simulink model "bipedal_robot_CTRL2"  (R2020b)
settings: Solver=ode23  StartTime=0.0  StopTime=Tsim  MaxStep=0.01  RelTol=1e-3  AbsTol=1e-3  EnableMultiTasking=on
values from neighbouring files (symbols this model uses):
  g = 9.80665    [bipedal.m]
  Tfil = Ts*10    (= 0.01)    [bipedal.m]
  total_mass = mlist(1) + ll_mass + rl_mass    [bipedal.m]
  Ts = 1/fs    (= 0.001)    [bipedal.m]
undefined symbols (not defined in the file or in its folder): Base, ctrl_cfg_rem, Fdist, LefAnklePitch, LefAnkleRoll, LefHipPitch, LefHipRoll, LefHipYaw, LefKnee, pg_traj, RigAnklePitch, RigAnkleRoll, RigHipPitch, RigHipRoll, RigHipYaw, RigKnee, sim_floor, Tdist, VAR_DIST, X, Y, Z
libraries: sm_lib x56, biped_lib x39, nesl_utility x18, simulink x3, Contact_Forces_Lib x2, robotmaniplib x1
(part 1 of 4)
settings Model: Creator=Andraž  LastModifiedBy=Andraž
settings SolverCC: AutoScaleAbsTol=off  ZeroCrossAlgorithm=Adaptive
settings DataIOCC: LimitDataPoints=on  MaxDataPoints=10000
settings OptimizationCC: DefaultParameterBehavior=Inlined  EnhancedBackFolding=on  PassReuseOutputArgsThreshold=0  OptimizeBlockOrder=speed  DifferentSizesBufferReuse=on  OptimizationCustomize=off
settings DebuggingCC: IgnoredZcDiagnostic=none  ParameterTunabilityLossMsg=error  AllowSymbolicDim=off  SFUnexpectedBacktrackingDiag=warning  SFNoUnconditionalDefaultTransitionDiag=warning  SFExecutionAtInitializationDiag=none  ArithmeticOperatorsInVariantConditions=warning
settings SFSimCC: SimCustomHeaderCode="#include \"magdwick.h\""  SimUserSources=magdwick.c  SimUseLocalCustomCode=off  CustomCodeUndefinedFunction=UseInterfaceOnly
settings RTWCC: RTWUseLocalCustomCode=off
settings CodeAppCC: ForceParamTrailComments=on  OperatorAnnotations=on
settings GRTTargetCC: TargetLangStandard=C89/C90 (ANSI)
settings ConfigComp: CovMetricSettings=dw  CovSaveCumulativeToWorkspaceVar=on  CovSaveSingleToWorkspaceVar=on  CovExternalEMLEnable=off  CovSFcnEnable=off
settings SimscapeCC: SimscapeLogType=all  SimscapeLogSimulationStatistics=on  SimscapeLogDataHistory=10000
settings DiagnosticsConfigSet: SimMechanicsRigidlyBoundBlock=none  SimMechanicsJointTargetOverSpecification=none
settings ExplorerConfigSet: InternalSimMechanicsExplorerSettings="<ExplorerConfiguration><canonicalview>default</canonicalview><AnimationSetting><BasePlaybackSpeed>1.0</BasePlaybackSpeed><PlaybackSpeedFactor>1.0</PlaybackSpeedFactor></AnimationSetting><TilePanel><TileInfo><Tiles Columns=\"1\" Count=\"1\" Rows=\"1\"><Column Weight=\"1\"/><Row Weight=\"1\"/><Tile Height=\"1\" Width=\"1\" X=\"0\" Y=\"0\"/></Tiles></TileInfo><SceneInfo><SceneViewer><BGColor><R>0.921568632125854492</R><G>0.913725495338439941</G><B>0.929411768913269043</B></BGColor><Camera><DoPerspective>off</DoPerspective><Position><X>1.46613297561511291</X><Y>0.0453876523198907741</Y><Z>0.392041392879294182</Z></Position><Center><X>-5.43948861508880555e-08</X><Y>0.0453876523198907741</Y><Z>0.392041392879294182</Z></Center><Up><X>-0</X><Y>0</Y><Z>1</Z></Up><ViewLimDist>1</ViewLimDist><YLim>0.627694802072910396</YLim><XLim>0.478013733886293257</XLim></Camera></SceneViewer></SceneInfo></TilePanel><MechEditorPanel><Cameras/><GfxPanelCameraMap/><VideoCreator><PlaybackSpeedRatio>1.0</PlaybackSpeedRatio><FrameRate>30</FrameRate><VideoFormat>Motion JPEG AVI</VideoFormat><FrameSize>auto</FrameSize></VideoCreator></MechEditorPanel></ExplorerConfiguration>"

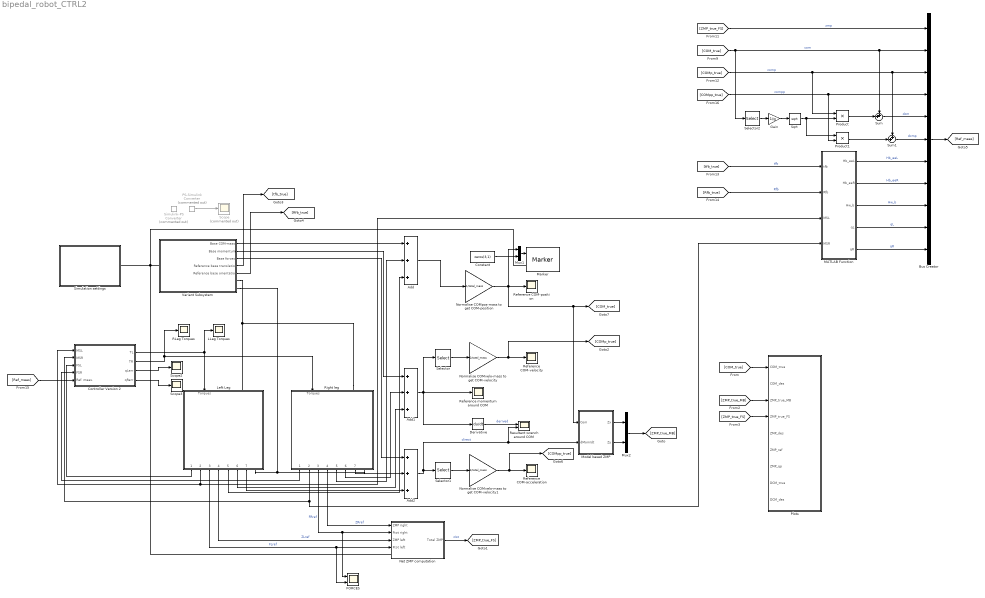
== system bipedal_robot_CTRL2 ==
  Add : Sum  Inputs=3
  Add1 : Sum  Inputs=3
  Add2 : Sum  Inputs=3
  Bus Creator : BusCreator  Inputs=11  OutDataTypeStr=Bus: meas_bus
  Constant : Constant  Value=zeros(3,1)
  Controller Version 2 : Subsystem  AncestorBlock=controller_lib/Controller Version 2  mask{ctrl_cfg_rem=ctrl_cfg_rem}
      mask prompts: ctrl_cfg_rem "Controller configuration structure"
  Derivative : Derivative  CoefficientInTFapproximation=400
  FORCES : Scope  NumInputPorts=2
  Gain : Gain  Gain=1/g
  LLeg Torques : Scope
  Left Leg : Subsystem
  MATLAB Function : MATLAB Function  TreatAsAtomicUnit=on  SystemSampleTime=Ts
  Marker : biped_lib/Marker  colour=[1.0 0.8 0.4]
  Model based ZMP : Subsystem  mask{M=total_mass, g=g, Tfil=Tfil*0.5}
      mask prompts: M "Mass"; g "Gravity"; Tfil "Filtering constant"
  Mux1 : Mux  Inputs=2
  Mux2 : Mux  Inputs=2
  Net ZMP computation : Subsystem
  Normalise COMpos-mass to get COM-position : Gain  Gain=1/total_mass
  Normalise COMvelo-mass to get COM-velocity : Gain  Gain=1/total_mass
  Normalise COMvelo-mass to get COM-velocity1 : Gain  Gain=1/total_mass
  PS-Simulink Converter : nesl_utility/PS-Simulink Converter  Commented=on  PhysicalDomain=network_engine_domain  SubClassName=ps_output  LeftPortType=input  RightPortType=output  PseudoPeriodic=off  Frequencies=[]  Unit=inherit  AffineConversion=off
      settings: SourceProductName=Utilities
  Plots : Subsystem
  Product : Product
  Product1 : Product
  RLeg Torques : Scope
  Reference COM-acceleration : Scope
  Reference COM-position : Scope
  Reference COM-velocity : Scope
  Reference momentum around COM : Scope
  Resultant wrench around COM : Scope  NumInputPorts=2
  Right leg : Subsystem
  Scope : Scope  Commented=on
  Scope2 : Scope
  Scope3 : Scope
  Selector : Selector  InputPortWidth=6  IndexOptions=Index vector (dialog)  Indices=[1 2 3]  OutputSizes=1
  Selector1 : Selector  InputPortWidth=6  IndexOptions=Index vector (dialog)  Indices=[1 2 3]  OutputSizes=1
  Selector2 : Selector  InputPortWidth=3  IndexOptions=Index vector (dialog)  Indices=[3]  OutputSizes=1
  Simulation settings : Subsystem
  Simulink-PS Converter : nesl_utility/Simulink-PS Converter  Commented=on  PhysicalDomain=network_engine_domain  SubClassName=ps_input  LeftPortType=input  RightPortType=output  PseudoPeriodic=off  Frequencies=[]  NoiseDistribution=none  NoiseParameters=[]  Unit=1  AffineConversion=off  FilteringAndDerivatives=provide  SimscapeFilterOrder=1  InputFilterTimeConstant=0.001  UdotUserProvided=0
      settings: SourceProductName=Utilities
  Sqrt : Sqrt  SaturateOnIntegerOverflow=on
  Sum : Sum  Inputs=++|
  Sum1 : Sum  Inputs=++|
  Variant Subsystem : Subsystem  Variant=on
  wires:
  PS-Simulink Converter/1 -> Scope/1
  Controller Version 2/1(TL) -> LLeg Torques/1, Left Leg/1(Torques)
  Controller Version 2/2(TR) -> Right leg/1(Torques), RLeg Torques/1
  Right leg/3(Total force) -> FORCES/1, Net ZMP computation/2(Ftot right)  "FRref"
  Left Leg/3(Total force) -> FORCES/2, Net ZMP computation/4(Ftot left)  "FLref"
  Right leg/4(Zero moment point) -> Net ZMP computation/1(ZMP right)  "ZRref"
  Left Leg/4(Zero moment point) -> Net ZMP computation/3(ZMP left)  "ZLref"
  Net ZMP computation/1(Total ZMP) -> [ZMP_true_FS]  "zIst"
  Left Leg/5(Leg COM-mass) -> Add/3
  Right leg/5(Leg COM-mass) -> Add/2
  Add/1 -> Normalise COMpos-mass to get COM-position/1
  Add1/1 -> Derivative/1, Reference momentum around COM/1, Selector/1
  Right leg/6(Leg momentum) -> Add1/2
  Left Leg/6(Leg momentum) -> Add1/3
  Derivative/1 -> Resultant wrench around COM/1  "derived"
  Selector/1 -> Normalise COMvelo-mass to get COM-velocity/1
  Normalise COMvelo-mass to get COM-velocity/1 -> [COMp_true], Reference COM-velocity/1
  Right leg/7(Leg momentum1) -> Add2/2
  Left Leg/7(Leg momentum1) -> Add2/3
  Add2/1 -> Selector1/1, Resultant wrench around COM/2, Model based ZMP/2(dMom/dt)  "direct"
  Normalise COMvelo-mass to get COM-velocity1/1 -> [COMpp_true], Reference COM-acceleration/1
  Selector1/1 -> Normalise COMvelo-mass to get COM-velocity1/1
  Normalise COMpos-mass to get COM-position/1 -> Mux1/1, Model based ZMP/1(Com), [COM_true], Reference COM-position/1
  Mux1/1 -> Marker/1
  Constant/1 -> Mux1/2
  Model based ZMP/1(Zx) -> Mux2/1
  Model based ZMP/2(Zy) -> Mux2/2
  Mux2/1 -> [ZMP_true_MB]
  [COM_true] -> Plots/1(COM_true)
  [ZMP_true_MB] -> Plots/3(ZMP_true_MB)
  [ZMP_true_FS] -> Plots/4(ZMP_true_FS)
  Left Leg/2(Motor sensory data) -> MATLAB Function/3(MSL), Controller Version 2/1(MSL)
  Right leg/2(Motor sensory data) -> MATLAB Function/4(MSR), Controller Version 2/2(MSR)
  Left Leg/1(Contact data) -> Controller Version 2/3(FSL)
  Right leg/1(Contact data) -> Controller Version 2/4(FSR)
  Controller Version 2/3(qLerr) -> Scope2/1
  Controller Version 2/4(qRerr) -> Scope3/1
  [COM_true] -> Selector2/1, Sum/1, Bus Creator/2  "com"
  Sum/1 -> Bus Creator/5  "dcm"
  [ZMP_true_FS] -> Bus Creator/1  "zmp"
  [COMp_true] -> Product/1, Bus Creator/3, Sum1/1  "comp"
  [tfb_true] -> MATLAB Function/1(tfb)  "tfb"
  [Rfb_true] -> MATLAB Function/2(Rfb)  "Rfb"
  Bus Creator/1 -> [Ref_meas]
  [Ref_meas] -> Controller Version 2/5(Ref. meas.)
  [COMpp_true] -> Product1/2, Bus Creator/4  "compp"
  Gain/1 -> Sqrt/1
  Selector2/1 -> Gain/1
  Sqrt/1 -> Product1/1, Product/2
  Product/1 -> Sum/2
  Product1/1 -> Sum1/2
  Sum1/1 -> Bus Creator/6  "dcmp"
  MATLAB Function/3(Hw_b) -> Bus Creator/9  "Hw_b"
  MATLAB Function/1(Hb_eeL) -> Bus Creator/7  "Hb_eeL"
  MATLAB Function/2(Hb_eeR) -> Bus Creator/8  "Hb_eeR"
  MATLAB Function/4(qL) -> Bus Creator/10  "qL"
  MATLAB Function/5(qR) -> Bus Creator/11  "qR"
  Variant Subsystem/1(Base COM-mass) -> Add/1
  Variant Subsystem/2(Base momentum) -> Add1/1
  Variant Subsystem/3(Base forces) -> Add2/1
  Variant Subsystem/4(Reference base translation) -> [tfb_true]
  Variant Subsystem/5(Reference base orientation) -> [Rfb_true]
  connections:
  Marker/LConn1 -- Simulation settings/RConn1 -- Variant Subsystem/LConn1 -- Net ZMP computation/LConn1
  Right leg/LConn1 -- Variant Subsystem/RConn1 -- Left Leg/LConn1
  Left Leg/RConn1 -- Right leg/RConn1 -- Variant Subsystem/RConn2

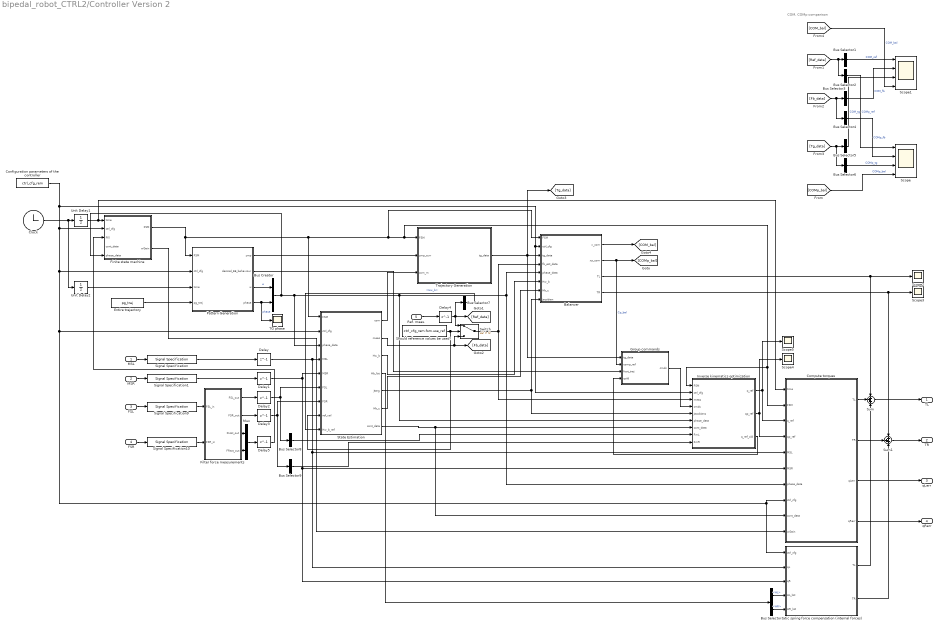
== system bipedal_robot_CTRL2/Controller Version 2 ==
  note: COM, COMp comparison
  MSL : Inport
  MSR : Inport  Port=2
  FSL : Inport  Port=3
  FSR : Inport  Port=4
  Ref. meas. : Inport  Port=5  OutDataTypeStr=Bus: meas_bus
  Balancer : MATLAB Function  TreatAsAtomicUnit=on
  Bus Creator : BusCreator  Inputs=2  OutDataTypeStr=Bus: ph_data_bus
  Bus Selector : BusSelector  OutputSignals=HL,HR
  Bus Selector1 : BusSelector  OutputSignals=com  OutputAsBus=on
  Bus Selector2 : BusSelector  OutputSignals=comp  OutputAsBus=on
  Bus Selector3 : BusSelector  OutputSignals=com  OutputAsBus=on
  Bus Selector4 : BusSelector  OutputSignals=comp  OutputAsBus=on
  Bus Selector5 : BusSelector  OutputSignals=com  OutputAsBus=on
  Bus Selector6 : BusSelector  OutputSignals=comp  OutputAsBus=on
  Bus Selector7 : BusSelector  OutputSignals=Hw_b
  Bus Selector8 : BusSelector  OutputSignals=Fm  OutputAsBus=on
  Bus Selector9 : BusSelector  OutputSignals=Fm  OutputAsBus=on
  Clock : Clock
  Compute torques : Subsystem
  Configuration parameters of the controller : Constant  Value=ctrl_cfg_rem  OutDataTypeStr=Bus: ctrl_cfg_rem_bus  SampleTime=ctrl_cfg_rem.par.Ts
  Delay : Delay  DelayLength=1  InitialCondition=ctrl_cfg_rem.fb_est.init.MSL  SampleTime=ctrl_cfg_rem.par.Ts
  Delay1 : Delay  DelayLength=1  InitialCondition=ctrl_cfg_rem.fb_est.init.MSR  SampleTime=ctrl_cfg_rem.par.Ts
  Delay2 : Delay  DelayLength=1  InitialCondition=ctrl_cfg_rem.fb_est.init.FSL  SampleTime=ctrl_cfg_rem.par.Ts
  Delay3 : Delay  DelayLength=1  InitialCondition=ctrl_cfg_rem.fb_est.init.FSR  SampleTime=ctrl_cfg_rem.par.Ts
  Delay4 : Delay  DelayLength=1  InitialCondition=0  SampleTime=ctrl_cfg_rem.par.Ts
  Delay5 : Delay  DelayLength=1  InitialCondition=[0;0]  SampleTime=ctrl_cfg_rem.par.Ts
  Entire trajectory : Constant  Value=pg_traj  VectorParams1D=off  OutDataTypeStr=Bus: pg_traj_bus  SampleTime=ctrl_cfg_rem.par.Ts
  Filter force measurements : Subsystem  mask{Tfil=ctrl_cfg_rem.fil.Tfil}
      mask prompts: Tfil "Filter T const"
  Finite state machine : MATLAB Function  TreatAsAtomicUnit=on
  Group commands : Subsystem
  Inverse kinematics optimization : Subsystem  Variant=on  mask{ik_opt=ctrl_cfg_rem.ik_opt, Ts=ctrl_cfg_rem.par.Ts}
      mask prompts: ik_opt "Ikine parameters"; Ts "Sampling time"
  Mux : Mux  Inputs=2
  Pattern Generation : Subsystem
  Scope : Scope  NumInputPorts=4
  Scope1 : Scope  NumInputPorts=4
  Scope{2..5} (4 alike) : Scope
  Should reference values be used? : Constant  Value=ctrl_cfg_rem.fsm.use_ref
  Signal Specification : SignalSpecification  OutDataTypeStr=Bus: leg_str_bus
  Signal Specification1 : SignalSpecification  OutDataTypeStr=Bus: leg_str_bus
  Signal Specification10 : SignalSpecification  OutDataTypeStr=Bus: fs_str_bus
  Signal Specification9 : SignalSpecification  OutDataTypeStr=Bus: fs_str_bus
  State Estimation : Subsystem  mask{fb_est=ctrl_cfg_rem.fb_est, Ts=ctrl_cfg_rem.par.Ts}
      mask prompts: fb_est "Floating base est. params"; Ts "Sampling time"
  Static spring force compensation (internal forces) : Subsystem
  Sum : Sum  Inputs=+++
  Sum1 : Sum  Inputs=+++
  Switch : Switch  Criteria=u2 > Threshold
  TG phase : Scope
  Trajectory Generation : Subsystem  Variant=on  mask{tg=ctrl_cfg_rem.tg}
      mask prompts: tg "Preview controller parameters"
  Unit Delay1 : UnitDelay  SampleTime=ctrl_cfg_rem.par.Ts  HasFrameUpgradeWarning=on
  Unit Delay2 : UnitDelay  SampleTime=ctrl_cfg_rem.par.Ts  HasFrameUpgradeWarning=on
  TL : Outport
  TR : Outport  Port=2
  qLerr : Outport  Port=3
  qRerr : Outport  Port=4
  wires:
  Compute torques/4(qRerr) -> qRerr/1
  Compute torques/3(qLerr) -> qLerr/1
  MSR/1 -> Signal Specification1/1
  FSL/1 -> Signal Specification9/1
  MSL/1 -> Signal Specification/1
  FSR/1 -> Signal Specification10/1
  Signal Specification1/1 -> Delay1/1
  Signal Specification/1 -> Delay/1
  Signal Specification9/1 -> Filter force measurements/1(FSL_in)
  Signal Specification10/1 -> Filter force measurements/2(FSR_in)
  Bus Selector/2 -> Static spring force compensation (internal forces)/5(HR_list)  "<HR>"
  Bus Selector/1 -> Static spring force compensation (internal forces)/4(HL_list)  "<HL>"
  Inverse kinematics optimization/3(q_ref_old) -> Group commands/4(qold)
  State Estimation/3(Hw_b) -> Balancer/6(Hw_b)
  Group commands/1(cmds) -> Inverse kinematics optimization/4(cmds)
  Pattern Generation/2(desired_EE_behaviour) -> Group commands/3(foot_traj)
  Trajectory Generation/1(tg_data) -> Group commands/1(tg_data), Balancer/3(tg_data), [Tg_data]
  Switch/1 -> Inverse kinematics optimization/3(meas), Balancer/4(fb_est_data)
  State Estimation/1(com) -> Trajectory Generation/3(com_m)
  Static spring force compensation (internal forces)/2(TR) -> Sum1/3
  Static spring force compensation (internal forces)/1(TL) -> Sum/3
  State Estimation/4(Hb_list) -> Bus Selector/1
  Compute torques/2(TR) -> Sum1/2
  Sum1/1 -> TR/1
  Sum/1 -> TL/1
  Compute torques/1(TL) -> Sum/2
  State Estimation/5(Jtarg) -> Balancer/8(jacobian), Inverse kinematics optimization/5(jacobians)
  Inverse kinematics optimization/2(qp_ref) -> Scope4/1, Compute torques/4(qp_ref)
  Inverse kinematics optimization/1(q_ref) -> Scope5/1, Compute torques/3(q_ref)
  Bus Creator/1 -> Finite state machine/5(phase_data), State Estimation/3(phase_data), Inverse kinematics optimization/6(phase_data), Balancer/5(phase_data), Compute torques/7(phase_data)
  Balancer/4(TR) -> Scope3/1, Sum1/1
  Balancer/3(TL) -> Scope2/1, Sum/1
  Pattern Generation/3(w) -> Bus Creator/1  "w"
  Delay2/1 -> State Estimation/6(FSL), Bus Selector8/1
  Unit Delay2/1 -> Pattern Generation/3(time)
  Finite state machine/1(FSM) -> Pattern Generation/1(FSM), Compute torques/2(FSM), Inverse kinematics optimization/1(FSM), Trajectory Generation/1(FSM), Balancer/1(FSM), State Estimation/1(FSM)
  Configuration parameters of the controller/1 -> Inverse kinematics optimization/2(ctrl_cfg), Balancer/2(ctrl_cfg), Pattern Generation/2(ctrl_cfg), State Estimation/2(ctrl_cfg), Static spring force compensation (internal forces)/1(ctrl_cfg), Compute torques/8(ctrl_cfg), Finite state machine/2(ctrl_cfg)
  Delay3/1 -> Bus Selector9/1, State Estimation/7(FSR)
  Delay1/1 -> State Estimation/5(MSR), Static spring force compensation (internal forces)/3(qR), Compute torques/6(MSR)
  Entire trajectory/1 -> Pattern Generation/4(pg_traj)
  Delay/1 -> Static spring force compensation (internal forces)/2(qL), Compute torques/5(MSL), State Estimation/4(MSL)
  Clock/1 -> Unit Delay2/1, Unit Delay1/1
  Unit Delay1/1 -> Compute torques/1(time), Finite state machine/1(time)
  Pattern Generation/4(phase) -> Bus Creator/2, TG phase/1  "phase"
  Pattern Generation/1(zmp) -> Trajectory Generation/2(zmp_curr)
  Balancer/2(xp_com) -> [COMp_bal], Group commands/2(comp_ref)  "Cp_bal"
  Ref. meas./1 -> Delay4/1
  Delay4/1 -> Bus Selector7/1, [Ref_data], Switch/1
  State Estimation/2(meas) -> [Fb_data], Switch/3
  Should reference values be used?/1 -> State Estimation/8(ref_val), Switch/2
  [Ref_data] -> Bus Selector2/1, Bus Selector1/1
  Bus Selector1/1 -> Scope1/1  "COM_ref"
  Bus Selector2/1 -> Scope/1  "COMp_ref"
  [Fb_data] -> Bus Selector4/1, Bus Selector3/1
  Bus Selector3/1 -> Scope1/2  "COM_fb"
  Bus Selector4/1 -> Scope/2  "COMp_fb"
  [COMp_bal] -> Scope/4  "COMp_bal"
  [Tg_data] -> Bus Selector6/1, Bus Selector5/1
  Bus Selector5/1 -> Scope1/3  "COM_tg"
  Bus Selector6/1 -> Scope/3  "COMp_tg"
  Balancer/1(x_com) -> [COM_bal]
  [COM_bal] -> Scope1/4  "COM_bal"
  Bus Selector7/1 -> State Estimation/9(Hw_b_ref)  "<Hw_b>"
  State Estimation/6(Hb_c) -> Balancer/7(Hb_c)
  Filter force measurements/1(FSL_out) -> Delay2/1
  Filter force measurements/2(FSR_out) -> Delay3/1
  Bus Selector8/1 -> Inverse kinematics optimization/8(FmL)
  Bus Selector9/1 -> Inverse kinematics optimization/9(FmR)
  Filter force measurements/4(FRtot_out) -> Mux/2
  Filter force measurements/3(FLtot_out) -> Mux/1
  Mux/1 -> Delay5/1
  State Estimation/7(cont_data) -> Compute torques/9(cont_data), Inverse kinematics optimization/7(cont_data)
  Delay5/1 -> Finite state machine/3(Ffil)
  Finite state machine/2(wGain) -> Compute torques/10(wGain)

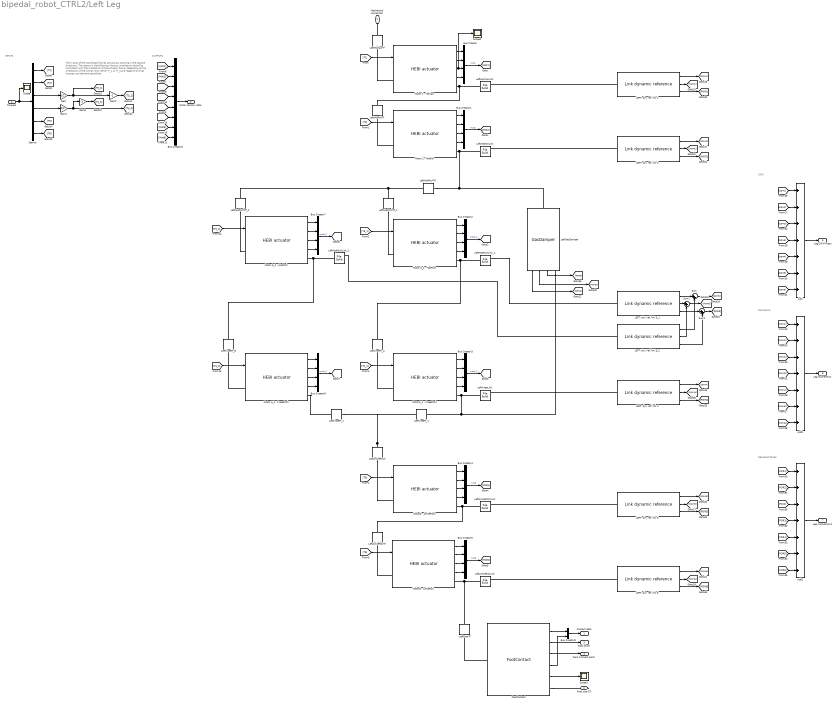
== system bipedal_robot_CTRL2/Left Leg ==
  note: Momentum
  note: COM
  note: OUTPUTS
  note: INPUTS
  note: The z-axes of the coordinate frames are always pointing in the
      | oposite directions. The reason is the following: the axis orientation
      | should be consistent with the orientation of the actuator frame. Depending on the orientation of the overall joint, either Ti_1 or Ti_2
      | are negative so that torques complement eachother
  note: Resultant forces
  Torques : Inport
  Add : Sum  Inputs=7
  Add1 : Sum  Inputs=7
  Add2 : Sum  Inputs=7
  Bus Creator{,1..5,7..8} (8 alike) : BusCreator  Inputs=4
  Bus Creator6 : BusCreator  Inputs=8  OutDataTypeStr=Bus: leg_str_bus
  Bus Creator9 : BusCreator  Inputs=2
  Demux : Demux  Outputs=6
  FootContact : biped_lib/FootContact  foot=foot  sim_floor=sim_floor  Ts=Ts
  Gain : Gain  Gain=1/2
  Gain1 : Gain  Gain=1/2
  Gain2 : Gain  Gain=-1
  Gain3 : Gain  Gain=-1
  LEFT: dyn. ref. link 1 : biped_lib/Link dynamic reference  M=LefHipYaw.body.com  I=LefHipYaw.body.inertia
  LEFT: dyn. ref. link 2 : biped_lib/Link dynamic reference  M=LefHipRoll.body.mass  I=LefHipRoll.body.inertia
  LEFT: dyn. ref. link 3_1 : biped_lib/Link dynamic reference  M=LefHipPitch.body.mass  I=LefHipPitch.body.inertia
  LEFT: dyn. ref. link 3_2 : biped_lib/Link dynamic reference  M=LefHipPitch.body.mass  I=LefHipPitch.body.inertia
  LEFT: dyn. ref. link 4 : biped_lib/Link dynamic reference  M=LefKnee.body.mass  I=LefKnee.body.inertia
  LEFT: dyn. ref. link 5 : biped_lib/Link dynamic reference  M=LefAnklePitch.body.mass  I=LefAnklePitch.body.inertia
  LEFT: dyn. ref. link 6 : biped_lib/Link dynamic reference  M=LefAnkleRoll.body.mass  I=LefAnkleRoll.body.inertia
  LeftAnklePitch : sm_lib/Frames and Transforms/Rigid Transform  TranslationMethod=Cartesian  TranslationStandardOffset=0  TranslationLengthUnit=m  TranslationStandardAxis=+Z  TranslationCartesianOffset=LefAnklePitch.pos  TranslationROffset=0  TranslationROffsetUnits=m  TranslationZOffset=0  TranslationZOffsetUnits=m  TranslationThetaOffset=0  TranslationThetaOffsetUnits=deg  RotationMethod=RotationSequence  RotationAngleUnits=deg  RotationStandardAxis=+Z  RotationAngle=0.0  RotationArbitraryAxis=[0 0 1]  FollAlignAxisA=+X  BaseAlignAxisA=+Y  FollAlignAxisB=+Y  BaseAlignAxisB=+Z  RotationSequenceAxes=FollowerAxes  RotationSequence=XYZ  RotationSequenceAngles=LefAnklePitch.rot  RotationSequenceAnglesUnits=rad  RotationMatrix=[1 0 0; 0 1 0; 0 0 1]
  LeftAnklePitchLink : sm_lib/Body Elements/File Solid  ExtGeomFileName=Link5L.stl  UnitType=Custom  ExtGeomFileUnits=mm  StepReaderType=HEX  ExportConvexHullGeometry=on  InertiaType=Custom  Mass=LefAnklePitch.body.mass  MassUnits=kg  CenterOfMass=LefAnklePitch.body.com  CenterOfMassUnits=m  MomentsOfInertia=LefAnklePitch.body.inertia(1:3)  MomentsOfInertiaUnits=kg*m^2  ProductsOfInertia=LefAnklePitch.body.inertia(4:6)  ProductsOfInertiaUnits=kg*m^2  BasedOnType=Mass  Density=1000  DensityUnits=kg/m^3  DoExposeReferenceFrame=on  SerializedFrames=<Frames><Frame><Id>Frame1</Id><Value><Name>COM</Name><Origin><Source>CenterOfMassFrame</Source><FeatureName></FeatureName></Origin><PrimaryAxis><DefinedDirection>+Z</DefinedDirection><Source>ReferenceFrame</Source><SourceDirection>+Z</SourceDirection><FeatureName></FeatureName></PrimaryAxis><SecondaryAxis><DefinedDirection>+X</DefinedDirection><Source>ReferenceFrame</Source><SourceDirection>+X</SourceDirection><FeatureName></FeatureName></SecondaryAxis></Value></Frame></Frames>  GraphicType=FromGeometry  MarkerShape=Sphere  MarkerSize=10  GraphicVisPropType=SimpleVisualProperties  GraphicDiffuseColor=[0.5 0.5 0.5]  GraphicSpecularColor=[0.5 0.5 0.5 1.0]  GraphicAmbientColor=[0.15 0.15 0.15 1.0]  GraphicEmissiveColor=[0.0 0.0 0.0 1.0]  GraphicShininess=75  GraphicOpacity=1.0
  LeftAnkleRollLink : sm_lib/Body Elements/File Solid  ExtGeomFileName=Link6.stl  UnitType=Custom  ExtGeomFileUnits=mm  StepReaderType=HEX  ExportConvexHullGeometry=on  InertiaType=Custom  Mass=LefAnkleRoll.body.mass  MassUnits=kg  CenterOfMass=LefAnkleRoll.body.com  CenterOfMassUnits=m  MomentsOfInertia=LefAnkleRoll.body.inertia(1:3)  MomentsOfInertiaUnits=kg*m^2  ProductsOfInertia=LefAnkleRoll.body.inertia(4:6)  ProductsOfInertiaUnits=kg*m^2  BasedOnType=Mass  Density=1000  DensityUnits=kg/m^3  DoExposeReferenceFrame=on  SerializedFrames=<Frames><Frame><Id>Frame1</Id><Value><Name>COM</Name><Origin><Source>CenterOfMassFrame</Source><FeatureName></FeatureName></Origin><PrimaryAxis><DefinedDirection>+Z</DefinedDirection><Source>ReferenceFrame</Source><SourceDirection>+Z</SourceDirection><FeatureName></FeatureName></PrimaryAxis><SecondaryAxis><DefinedDirection>+X</DefinedDirection><Source>ReferenceFrame</Source><SourceDirection>+X</SourceDirection><FeatureName></FeatureName></SecondaryAxis></Value></Frame></Frames>  GraphicType=FromGeometry  MarkerShape=Sphere  MarkerSize=10  GraphicVisPropType=SimpleVisualProperties  GraphicDiffuseColor=[0.5 0.5 0.5]  GraphicSpecularColor=[0.5 0.5 0.5 1.0]  GraphicAmbientColor=[0.15 0.15 0.15 1.0]  GraphicEmissiveColor=[0.0 0.0 0.0 1.0]  GraphicShininess=75  GraphicOpacity=1.0
  LeftAnkleRollTf : sm_lib/Frames and Transforms/Rigid Transform  TranslationMethod=Cartesian  TranslationStandardOffset=0  TranslationLengthUnit=m  TranslationStandardAxis=+Z  TranslationCartesianOffset=LefAnkleRoll.pos  TranslationROffset=0  TranslationROffsetUnits=m  TranslationZOffset=0  TranslationZOffsetUnits=m  TranslationThetaOffset=0  TranslationThetaOffsetUnits=deg  RotationMethod=RotationSequence  RotationAngleUnits=deg  RotationStandardAxis=+Z  RotationAngle=0.0  RotationArbitraryAxis=[0 0 1]  FollAlignAxisA=+Z  BaseAlignAxisA=+X  FollAlignAxisB=+Y  BaseAlignAxisB=+Y  RotationSequenceAxes=FollowerAxes  RotationSequence=XYZ  RotationSequenceAngles=LefAnkleRoll.rot  RotationSequenceAnglesUnits=rad  RotationMatrix=[1 0 0; 0 1 0; 0 0 1]
  LeftFootTf : sm_lib/Frames and Transforms/Rigid Transform  TranslationMethod=Cartesian  TranslationStandardOffset=0  TranslationLengthUnit=m  TranslationStandardAxis=+Z  TranslationCartesianOffset=LefFoot.pos  TranslationROffset=0  TranslationROffsetUnits=m  TranslationZOffset=0  TranslationZOffsetUnits=m  TranslationThetaOffset=0  TranslationThetaOffsetUnits=deg  RotationMethod=RotationSequence  RotationAngleUnits=deg  RotationStandardAxis=+Z  RotationAngle=0.0  RotationArbitraryAxis=[0 0 1]  FollAlignAxisA=+Z  BaseAlignAxisA=+Y  FollAlignAxisB=+X  BaseAlignAxisB=+X  RotationSequenceAxes=FollowerAxes  RotationSequence=XYZ  RotationSequenceAngles=LefFoot.rot  RotationSequenceAnglesUnits=rad  RotationMatrix=[1 0 0; 0 1 0; 0 0 1]
  LeftGasDamper : biped_lib/GasDamper  mech=LefDamper
  LeftHipPitchLink_1 : sm_lib/Body Elements/File Solid  ExtGeomFileName=Link3.stl  UnitType=Custom  ExtGeomFileUnits=mm  StepReaderType=HEX  ExportConvexHullGeometry=on  InertiaType=Custom  Mass=LefHipPitch.body.mass  MassUnits=kg  CenterOfMass=LefHipPitch.body.com  CenterOfMassUnits=m  MomentsOfInertia=LefHipPitch.body.inertia(1:3)  MomentsOfInertiaUnits=kg*m^2  ProductsOfInertia=LefHipPitch.body.inertia(4:6)  ProductsOfInertiaUnits=kg*m^2  BasedOnType=Mass  Density=1000  DensityUnits=kg/m^3  DoExposeReferenceFrame=on  SerializedFrames=<Frames><Frame><Id>Frame1</Id><Value><Name>COM</Name><Origin><Source>CenterOfMassFrame</Source><FeatureName></FeatureName></Origin><PrimaryAxis><DefinedDirection>+Z</DefinedDirection><Source>ReferenceFrame</Source><SourceDirection>+Z</SourceDirection><FeatureName></FeatureName></PrimaryAxis><SecondaryAxis><DefinedDirection>+X</DefinedDirection><Source>ReferenceFrame</Source><SourceDirection>+X</SourceDirection><FeatureName></FeatureName></SecondaryAxis></Value></Frame></Frames>  GraphicType=FromGeometry  MarkerShape=Sphere  MarkerSize=10  GraphicVisPropType=SimpleVisualProperties  GraphicDiffuseColor=[0.5 0.5 0.5]  GraphicSpecularColor=[0.5 0.5 0.5 1.0]  GraphicAmbientColor=[0.15 0.15 0.15 1.0]  GraphicEmissiveColor=[0.0 0.0 0.0 1.0]  GraphicShininess=75  GraphicOpacity=1.0
  LeftHipPitchLink_2 : sm_lib/Body Elements/File Solid  ExtGeomFileName=Link3.stl  UnitType=Custom  ExtGeomFileUnits=mm  StepReaderType=HEX  ExportConvexHullGeometry=on  InertiaType=Custom  Mass=LefHipPitch.body.mass  MassUnits=kg  CenterOfMass=LefHipPitch.body.com  CenterOfMassUnits=m  MomentsOfInertia=LefHipPitch.body.inertia(1:3)  MomentsOfInertiaUnits=kg*m^2  ProductsOfInertia=LefHipPitch.body.inertia(4:6)  ProductsOfInertiaUnits=kg*m^2  BasedOnType=Mass  Density=1000  DensityUnits=kg/m^3  DoExposeReferenceFrame=on  SerializedFrames=<Frames><Frame><Id>Frame1</Id><Value><Name>COM</Name><Origin><Source>CenterOfMassFrame</Source><FeatureName></FeatureName></Origin><PrimaryAxis><DefinedDirection>+Z</DefinedDirection><Source>ReferenceFrame</Source><SourceDirection>+Z</SourceDirection><FeatureName></FeatureName></PrimaryAxis><SecondaryAxis><DefinedDirection>+X</DefinedDirection><Source>ReferenceFrame</Source><SourceDirection>+X</SourceDirection><FeatureName></FeatureName></SecondaryAxis></Value></Frame></Frames>  GraphicType=FromGeometry  MarkerShape=Sphere  MarkerSize=10  GraphicVisPropType=SimpleVisualProperties  GraphicDiffuseColor=[0.5 0.5 0.5]  GraphicSpecularColor=[0.5 0.5 0.5 1.0]  GraphicAmbientColor=[0.15 0.15 0.15 1.0]  GraphicEmissiveColor=[0.0 0.0 0.0 1.0]  GraphicShininess=75  GraphicOpacity=1.0
  LeftHipPitchTf : sm_lib/Frames and Transforms/Rigid Transform  TranslationMethod=Cartesian  TranslationStandardOffset=0  TranslationLengthUnit=m  TranslationStandardAxis=+Z  TranslationCartesianOffset=LefHipPitch.pos  TranslationROffset=0  TranslationROffsetUnits=m  TranslationZOffset=0  TranslationZOffsetUnits=m  TranslationThetaOffset=0  TranslationThetaOffsetUnits=deg  RotationMethod=RotationSequence  RotationAngleUnits=deg  RotationStandardAxis=+Z  RotationAngle=0.0  RotationArbitraryAxis=[0 0 1]  FollAlignAxisA=+Z  BaseAlignAxisA=-X  FollAlignAxisB=+Y  BaseAlignAxisB=+Y  RotationSequenceAxes=FollowerAxes  RotationSequence=XYZ  RotationSequenceAngles=LefHipPitch.rot  RotationSequenceAnglesUnits=rad  RotationMatrix=[1 0 0; 0 1 0; 0 0 1]
  LeftHipPitchTf_1 : sm_lib/Frames and Transforms/Rigid Transform  TranslationMethod=Cartesian  TranslationStandardOffset=0  TranslationLengthUnit=m  TranslationStandardAxis=+Z  TranslationCartesianOffset=LefHipPitch.pos_1  TranslationROffset=0  TranslationROffsetUnits=m  TranslationZOffset=0  TranslationZOffsetUnits=m  TranslationThetaOffset=0  TranslationThetaOffsetUnits=deg  RotationMethod=RotationSequence  RotationAngleUnits=deg  RotationStandardAxis=+Z  RotationAngle=0.0  RotationArbitraryAxis=[0 0 1]  FollAlignAxisA=+X  BaseAlignAxisA=+Y  FollAlignAxisB=+Y  BaseAlignAxisB=+Z  RotationSequenceAxes=FollowerAxes  RotationSequence=XYZ  RotationSequenceAngles=LefHipPitch.rot_1  RotationSequenceAnglesUnits=rad  RotationMatrix=[1 0 0; 0 1 0; 0 0 1]
  LeftHipPitchTf_2 : sm_lib/Frames and Transforms/Rigid Transform  TranslationMethod=Cartesian  TranslationStandardOffset=0  TranslationLengthUnit=m  TranslationStandardAxis=+Z  TranslationCartesianOffset=LefHipPitch.pos_2  TranslationROffset=0  TranslationROffsetUnits=m  TranslationZOffset=0  TranslationZOffsetUnits=m  TranslationThetaOffset=0  TranslationThetaOffsetUnits=deg  RotationMethod=RotationSequence  RotationAngleUnits=deg  RotationStandardAxis=+Z  RotationAngle=0.0  RotationArbitraryAxis=[0 0 1]  FollAlignAxisA=+X  BaseAlignAxisA=+Y  FollAlignAxisB=+Y  BaseAlignAxisB=+Z  RotationSequenceAxes=FollowerAxes  RotationSequence=XYZ  RotationSequenceAngles=LefHipPitch.rot_2  RotationSequenceAnglesUnits=rad  RotationMatrix=[1 0 0; 0 1 0; 0 0 1]
  LeftHipRollLink : sm_lib/Body Elements/File Solid  ExtGeomFileName=Link2.stl  UnitType=Custom  ExtGeomFileUnits=mm  StepReaderType=HEX  ExportConvexHullGeometry=on  InertiaType=Custom  Mass=LefHipRoll.body.mass  MassUnits=kg  CenterOfMass=LefHipRoll.body.com  CenterOfMassUnits=m  MomentsOfInertia=LefHipRoll.body.inertia(1:3)  MomentsOfInertiaUnits=kg*m^2  ProductsOfInertia=LefHipRoll.body.inertia(4:6)  ProductsOfInertiaUnits=kg*m^2  BasedOnType=Mass  Density=1000  DensityUnits=kg/m^3  DoExposeReferenceFrame=on  SerializedFrames=<Frames><Frame><Id>Frame1</Id><Value><Name>COM</Name><Origin><Source>CenterOfMassFrame</Source><FeatureName></FeatureName></Origin><PrimaryAxis><DefinedDirection>+Z</DefinedDirection><Source>ReferenceFrame</Source><SourceDirection>+Z</SourceDirection><FeatureName></FeatureName></PrimaryAxis><SecondaryAxis><DefinedDirection>+X</DefinedDirection><Source>ReferenceFrame</Source><SourceDirection>+X</SourceDirection><FeatureName></FeatureName></SecondaryAxis></Value></Frame></Frames>  GraphicType=FromGeometry  MarkerShape=Sphere  MarkerSize=10  GraphicVisPropType=SimpleVisualProperties  GraphicDiffuseColor=[0.5 0.5 0.5]  GraphicSpecularColor=[0.5 0.5 0.5 1.0]  GraphicAmbientColor=[0.15 0.15 0.15 1.0]  GraphicEmissiveColor=[0.0 0.0 0.0 1.0]  GraphicShininess=75  GraphicOpacity=1.0
  LeftHipRollTf : sm_lib/Frames and Transforms/Rigid Transform  TranslationMethod=Cartesian  TranslationStandardOffset=0  TranslationLengthUnit=m  TranslationStandardAxis=+Z  TranslationCartesianOffset=LefHipRoll.pos  TranslationROffset=0  TranslationROffsetUnits=m  TranslationZOffset=0  TranslationZOffsetUnits=m  TranslationThetaOffset=0  TranslationThetaOffsetUnits=deg  RotationMethod=RotationSequence  RotationAngleUnits=deg  RotationStandardAxis=+Z  RotationAngle=0.0  RotationArbitraryAxis=[0 0 1]  FollAlignAxisA=+Z  BaseAlignAxisA=+Y  FollAlignAxisB=+X  BaseAlignAxisB=+X  RotationSequenceAxes=FollowerAxes  RotationSequence=XYZ  RotationSequenceAngles=LefHipRoll.rot  RotationSequenceAnglesUnits=rad  RotationMatrix=[1 0 0; 0 1 0; 0 0 1]
  LeftHipYawLink : sm_lib/Body Elements/File Solid  ExtGeomFileName=Link1L.stl  UnitType=Custom  ExtGeomFileUnits=mm  StepReaderType=HEX  ExportConvexHullGeometry=on  InertiaType=Custom  Mass=LefHipYaw.body.mass  MassUnits=kg  CenterOfMass=LefHipYaw.body.com  CenterOfMassUnits=m  MomentsOfInertia=LefHipYaw.body.inertia(1:3)  MomentsOfInertiaUnits=kg*m^2  ProductsOfInertia=LefHipYaw.body.inertia(4:6)  ProductsOfInertiaUnits=kg*m^2  BasedOnType=Mass  Density=1000  DensityUnits=kg/m^3  DoExposeReferenceFrame=on  SerializedFrames=<Frames><Frame><Id>Frame1</Id><Value><Name>COM</Name><Origin><Source>CenterOfMassFrame</Source><FeatureName></FeatureName></Origin><PrimaryAxis><DefinedDirection>+Z</DefinedDirection><Source>ReferenceFrame</Source><SourceDirection>+Z</SourceDirection><FeatureName></FeatureName></PrimaryAxis><SecondaryAxis><DefinedDirection>+X</DefinedDirection><Source>ReferenceFrame</Source><SourceDirection>+X</SourceDirection><FeatureName></FeatureName></SecondaryAxis></Value></Frame></Frames>  GraphicType=FromGeometry  MarkerShape=Sphere  MarkerSize=10  GraphicVisPropType=SimpleVisualProperties  GraphicDiffuseColor=[0.5 0.5 0.5]  GraphicSpecularColor=[0.5 0.5 0.5 1.0]  GraphicAmbientColor=[0.15 0.15 0.15 1.0]  GraphicEmissiveColor=[0.0 0.0 0.0 1.0]  GraphicShininess=75  GraphicOpacity=1.0
  LeftHipYawTf : sm_lib/Frames and Transforms/Rigid Transform  TranslationMethod=Cartesian  TranslationStandardOffset=0  TranslationLengthUnit=m  TranslationStandardAxis=+Z  TranslationCartesianOffset=LefHipYaw.pos  TranslationROffset=0  TranslationROffsetUnits=m  TranslationZOffset=0  TranslationZOffsetUnits=m  TranslationThetaOffset=0  TranslationThetaOffsetUnits=deg  RotationMethod=RotationSequence  RotationAngleUnits=deg  RotationStandardAxis=+Z  RotationAngle=0.0  RotationArbitraryAxis=[0 0 1]  FollAlignAxisA=+X  BaseAlignAxisA=+Y  FollAlignAxisB=+Y  BaseAlignAxisB=+Z  RotationSequenceAxes=FollowerAxes  RotationSequence=XYZ  RotationSequenceAngles=LefHipYaw.rot  RotationSequenceAnglesUnits=rad  RotationMatrix=[1 0 0; 0 1 0; 0 0 1]
  LeftKneeLink : sm_lib/Body Elements/File Solid  ExtGeomFileName=Link4.stl  UnitType=Custom  ExtGeomFileUnits=mm  StepReaderType=HEX  ExportConvexHullGeometry=on  InertiaType=Custom  Mass=LefKnee.body.mass  MassUnits=kg  CenterOfMass=LefKnee.body.com  CenterOfMassUnits=m  MomentsOfInertia=LefKnee.body.inertia(1:3)  MomentsOfInertiaUnits=kg*m^2  ProductsOfInertia=LefKnee.body.inertia(4:6)  ProductsOfInertiaUnits=kg*m^2  BasedOnType=Mass  Density=1000  DensityUnits=kg/m^3  DoExposeReferenceFrame=on  SerializedFrames=<Frames><Frame><Id>Frame1</Id><Value><Name>COM</Name><Origin><Source>CenterOfMassFrame</Source><FeatureName></FeatureName></Origin><PrimaryAxis><DefinedDirection>+Z</DefinedDirection><Source>ReferenceFrame</Source><SourceDirection>+Z</SourceDirection><FeatureName></FeatureName></PrimaryAxis><SecondaryAxis><DefinedDirection>+X</DefinedDirection><Source>ReferenceFrame</Source><SourceDirection>+X</SourceDirection><FeatureName></FeatureName></SecondaryAxis></Value></Frame></Frames>  GraphicType=FromGeometry  MarkerShape=Sphere  MarkerSize=10  GraphicVisPropType=SimpleVisualProperties  GraphicDiffuseColor=[0.5 0.5 0.5]  GraphicSpecularColor=[0.5 0.5 0.5 1.0]  GraphicAmbientColor=[0.15 0.15 0.15 1.0]  GraphicEmissiveColor=[0.0 0.0 0.0 1.0]  GraphicShininess=75  GraphicOpacity=1.0
  LeftKneeTf_1 : sm_lib/Frames and Transforms/Rigid Transform  TranslationMethod=Cartesian  TranslationStandardOffset=0  TranslationLengthUnit=m  TranslationStandardAxis=+Z  TranslationCartesianOffset=LefKnee.pos_1  TranslationROffset=0  TranslationROffsetUnits=m  TranslationZOffset=0  TranslationZOffsetUnits=m  TranslationThetaOffset=0  TranslationThetaOffsetUnits=deg  RotationMethod=RotationSequence  RotationAngleUnits=deg  RotationStandardAxis=+Z  RotationAngle=0.0  RotationArbitraryAxis=[0 0 1]  FollAlignAxisA=+X  BaseAlignAxisA=+Y  FollAlignAxisB=+Y  BaseAlignAxisB=+Z  RotationSequenceAxes=FollowerAxes  RotationSequence=XYZ  RotationSequenceAngles=LefKnee.rot_1  RotationSequenceAnglesUnits=rad  RotationMatrix=[1 0 0; 0 1 0; 0 0 1]
  LeftKneeTf_2 : sm_lib/Frames and Transforms/Rigid Transform  TranslationMethod=Cartesian  TranslationStandardOffset=0  TranslationLengthUnit=m  TranslationStandardAxis=+Z  TranslationCartesianOffset=LefKnee.pos_2  TranslationROffset=0  TranslationROffsetUnits=m  TranslationZOffset=0  TranslationZOffsetUnits=m  TranslationThetaOffset=0  TranslationThetaOffsetUnits=deg  RotationMethod=RotationSequence  RotationAngleUnits=deg  RotationStandardAxis=+Z  RotationAngle=0.0  RotationArbitraryAxis=[0 0 1]  FollAlignAxisA=+X  BaseAlignAxisA=+Y  FollAlignAxisB=+Y  BaseAlignAxisB=+Z  RotationSequenceAxes=FollowerAxes  RotationSequence=XYZ  RotationSequenceAngles=LefKnee.rot_2  RotationSequenceAnglesUnits=rad  RotationMatrix=[1 0 0; 0 1 0; 0 0 1]
  LeftKneeTf_A : sm_lib/Frames and Transforms/Rigid Transform  TranslationMethod=Cartesian  TranslationStandardOffset=0  TranslationLengthUnit=m  TranslationStandardAxis=+Z  TranslationCartesianOffset=LefKnee.pos  TranslationROffset=0  TranslationROffsetUnits=m  TranslationZOffset=0  TranslationZOffsetUnits=m  TranslationThetaOffset=0  TranslationThetaOffsetUnits=deg  RotationMethod=RotationSequence  RotationAngleUnits=deg  RotationStandardAxis=+Z  RotationAngle=0.0  RotationArbitraryAxis=[0 0 1]  FollAlignAxisA=+X  BaseAlignAxisA=+Y  FollAlignAxisB=+Y  BaseAlignAxisB=+Z  RotationSequenceAxes=FollowerAxes  RotationSequence=XYZ  RotationSequenceAngles=LefKnee.rot  RotationSequenceAnglesUnits=rad  RotationMatrix=[1 0 0; 0 1 0; 0 0 1]
  LeftKneeTf_B : sm_lib/Frames and Transforms/Rigid Transform  TranslationMethod=Cartesian  TranslationStandardOffset=0  TranslationLengthUnit=m  TranslationStandardAxis=+Z  TranslationCartesianOffset=LefKnee.pos  TranslationROffset=0  TranslationROffsetUnits=m  TranslationZOffset=0  TranslationZOffsetUnits=m  TranslationThetaOffset=0  TranslationThetaOffsetUnits=deg  RotationMethod=RotationSequence  RotationAngleUnits=deg  RotationStandardAxis=+Z  RotationAngle=0.0  RotationArbitraryAxis=[0 0 1]  FollAlignAxisA=+X  BaseAlignAxisA=+Y  FollAlignAxisB=+Y  BaseAlignAxisB=+Z  RotationSequenceAxes=FollowerAxes  RotationSequence=XYZ  RotationSequenceAngles=LefKnee.rot  RotationSequenceAnglesUnits=rad  RotationMatrix=[1 0 0; 0 1 0; 0 0 1]
  Motor 1 - HipYaw : biped_lib/HEBI actuator  Tmax=motor.X8.v16.Tmax  qinit=LefHipYaw.qinit  IMU=LefHipYaw.IMU
  Motor 2 - HipRoll : biped_lib/HEBI actuator  Tmax=motor.X8.v16.Tmax  qinit=LefHipRoll.qinit  IMU=LefHipRoll.IMU
  Motor 3_1 - HipPitch : biped_lib/HEBI actuator  Tmax=motor.X8.v16.Tmax  qinit=LefHipPitch.qinit_1  IMU=LefHipPitch.IMU_1
  Motor 3_2 - HipPitch : biped_lib/HEBI actuator  Tmax=motor.X8.v16.Tmax  qinit=LefHipPitch.qinit_2  IMU=LefHipPitch.IMU_2
  Motor 4_2 - KneePitch : biped_lib/HEBI actuator  Tmax=motor.X8.v16.Tmax  qinit=LefKnee.qinit_2  IMU=LefKnee.IMU_2
  Motor4_1 - KneePitch : biped_lib/HEBI actuator  Tmax=motor.X8.v16.Tmax  qinit=LefKnee.qinit_1  IMU=LefKnee.IMU_1
  Motor5 - AnklePitch : biped_lib/HEBI actuator  Tmax=motor.X8.v16.Tmax  qinit=LefAnklePitch.qinit  IMU=LefAnklePitch.IMU
  Motor6 - AnkleRoll : biped_lib/HEBI actuator  Tmax=motor.X8.v16.Tmax  qinit=LefAnkleRoll.qinit  IMU=LefAnkleRoll.IMU
  Scope : Scope
  Scope1 : Scope
  Scope2 : Scope
  Sum : Sum  Inputs=|++
  Sum1 : Sum  Inputs=|++
  Sum2 : Sum  Inputs=|++
  Mechanical connection : PMIOPort  Side=Left
  Foot sole CF : PMIOPort  Port=2  Side=Right
  Contact data : Outport
  Motor sensory data : Outport  Port=2
  Total force : Outport  Port=3
  Zero moment point : Outport  Port=4
  Leg COM-mass : Outport  Port=5
  Leg momentum : Outport  Port=6
  Leg momentum1 : Outport  Port=7
  wires:
  FootContact/1 -> Bus Creator9/1
  Motor 1 - HipYaw/4 -> Bus Creator/4
  Motor 1 - HipYaw/3 -> Scope2/1, Bus Creator/3
  Motor 1 - HipYaw/2 -> Bus Creator/2
  Motor 1 - HipYaw/1 -> Bus Creator/1
  Motor 2 - HipRoll/1 -> Bus Creator1/1
  Motor 2 - HipRoll/2 -> Bus Creator1/2
  Motor 2 - HipRoll/3 -> Bus Creator1/3
  Motor 2 - HipRoll/4 -> Bus Creator1/4
  Motor 3_1 - HipPitch/2 -> Bus Creator2/2
  Motor 3_1 - HipPitch/1 -> Bus Creator2/1
  Motor 3_1 - HipPitch/3 -> Bus Creator2/3
  Motor 3_1 - HipPitch/4 -> Bus Creator2/4
  Motor4_1 - KneePitch/1 -> Bus Creator3/1
  Motor4_1 - KneePitch/2 -> Bus Creator3/2
  Motor4_1 - KneePitch/3 -> Bus Creator3/3
  Motor4_1 - KneePitch/4 -> Bus Creator3/4
  Motor5 - AnklePitch/1 -> Bus Creator4/1
  Motor5 - AnklePitch/2 -> Bus Creator4/2
  Motor5 - AnklePitch/3 -> Bus Creator4/3
  Motor5 - AnklePitch/4 -> Bus Creator4/4
  Motor6 - AnkleRoll/1 -> Bus Creator5/1
  Motor6 - AnkleRoll/2 -> Bus Creator5/2
  Motor6 - AnkleRoll/3 -> Bus Creator5/3
  Motor6 - AnkleRoll/4 -> Bus Creator5/4
  [T1] -> Motor 1 - HipYaw/1
  [T2] -> Motor 2 - HipRoll/1
  [T3_1] -> Motor 3_1 - HipPitch/1
  [T4_1] -> Motor4_1 - KneePitch/1
  [T5] -> Motor5 - AnklePitch/1
  [T6] -> Motor6 - AnkleRoll/1
  Bus Creator/1 -> [Mot1]  "mot1"
  Bus Creator1/1 -> [Mot2]  "mot2"
  Bus Creator2/1 -> [Mot3_1]  "mot3_1"
  Bus Creator3/1 -> [Mot4_1]  "mot4_1"
  Bus Creator4/1 -> [Mot5]  "mot5"
  Bus Creator5/1 -> [Mot6]  "mot6"
  Bus Creator6/1 -> Motor sensory data/1
  [Mot1] -> Bus Creator6/1
  [Mot2] -> Bus Creator6/2
  [Mot3_1] -> Bus Creator6/3
  [Mot4_1] -> Bus Creator6/5
  [Mot5] -> Bus Creator6/7
  [Mot6] -> Bus Creator6/8
  [Mot3_2] -> Bus Creator6/4
  [Mot4_2] -> Bus Creator6/6
  Bus Creator7/1 -> [Mot3_2]  "mot3_2"
  Motor 3_2 - HipPitch/2 -> Bus Creator7/2
  [T3_2] -> Motor 3_2 - HipPitch/1
  Motor 3_2 - HipPitch/1 -> Bus Creator7/1
  Motor 3_2 - HipPitch/3 -> Bus Creator7/3
  Motor 3_2 - HipPitch/4 -> Bus Creator7/4
  Bus Creator8/1 -> [Mot4_2]  "mot4_2"
  Motor 4_2 - KneePitch/3 -> Bus Creator8/3
  Motor 4_2 - KneePitch/2 -> Bus Creator8/2
  [T4_2] -> Motor 4_2 - KneePitch/1
  Motor 4_2 - KneePitch/4 -> Bus Creator8/4
  Motor 4_2 - KneePitch/1 -> Bus Creator8/1
  Torques/1 -> Scope/1, Demux/1
  Demux/1 -> [T1]
  Demux/2 -> [T2]
  Demux/3 -> Gain/1
  Gain/1 -> Gain2/1, [T3_1]
  Gain1/1 -> Gain3/1, [T4_2]
  Demux/4 -> Gain1/1
  Gain2/1 -> [T3_2]
  Gain3/1 -> [T4_1]
  Demux/5 -> [T5]
  Demux/6 -> [T6]
  FootContact/4 -> Bus Creator9/2
  Bus Creator9/1 -> Contact data/1
  FootContact/2 -> Total force/1
  FootContact/3 -> Zero moment point/1
  Add/1 -> Leg COM-mass/1
  Add1/1 -> Leg momentum/1
  LEFT: dyn. ref. link 1/1 -> [COM1]
  [COM1] -> Add/1
  LEFT: dyn. ref. link 2/1 -> [COM2]
  [COM2] -> Add/2
  [COM3] -> Add/4
  [COM4] -> Add/5
  [COM5] -> Add/6
  [COM6] -> Add/7
  [COMD] -> Add/3
  LEFT: dyn. ref. link 4/1 -> [COM4]
  LEFT: dyn. ref. link 5/1 -> [COM5]
  LEFT: dyn. ref. link 6/1 -> [COM6]
  LeftGasDamper/1 -> [COMD]
  LEFT: dyn. ref. link 1/2 -> [MOM1]
  LEFT: dyn. ref. link 2/2 -> [MOM2]
  LEFT: dyn. ref. link 4/2 -> [MOM4]
  LEFT: dyn. ref. link 5/2 -> [MOM5]
  LEFT: dyn. ref. link 6/2 -> [MOM6]
  LeftGasDamper/2 -> [MOMD]
  [MOM3] -> Add1/4
  [MOM5] -> Add1/6
  [MOM1] -> Add1/1
  [MOM6] -> Add1/7
  [MOM2] -> Add1/2
  [MOMD] -> Add1/3
  [MOM4] -> Add1/5
  [FOR2] -> Add2/2
  [FOR4] -> Add2/5
  [FOR6] -> Add2/7
  [FOR3] -> Add2/4
  [FORD] -> Add2/3
  [FOR5] -> Add2/6
  Add2/1 -> Leg momentum1/1
  [FOR1] -> Add2/1
  LEFT: dyn. ref. link 1/3 -> [FOR1]
  LEFT: dyn. ref. link 2/3 -> [FOR2]
  LEFT: dyn. ref. link 4/3 -> [FOR4]
  LEFT: dyn. ref. link 5/3 -> [FOR5]
  LEFT: dyn. ref. link 6/3 -> [FOR6]
  LeftGasDamper/3 -> [FORD]
  FootContact/5 -> Scope1/1
  Sum1/1 -> [MOM3]
  Sum/1 -> [COM3]
  Sum2/1 -> [FOR3]
  LEFT: dyn. ref. link 3_1/1 -> Sum/1
  LEFT: dyn. ref. link 3_2/1 -> Sum/2
  LEFT: dyn. ref. link 3_1/2 -> Sum1/1
  LEFT: dyn. ref. link 3_2/2 -> Sum1/2
  LEFT: dyn. ref. link 3_2/3 -> Sum2/2
  LEFT: dyn. ref. link 3_1/3 -> Sum2/1
  connections:
  LeftHipPitchTf/RConn1 -- LeftHipPitchTf_2/LConn1 -- LeftHipPitchTf_1/LConn1
  Motor6 - AnkleRoll/LConn1 -- LeftAnkleRollTf/RConn1
  Motor 2 - HipRoll/LConn1 -- LeftHipRollTf/RConn1
  LeftAnkleRollTf/LConn1 -- Motor5 - AnklePitch/RConn1 -- LeftAnklePitchLink/RConn1
  LeftHipPitchTf/LConn1 -- LeftGasDamper/LConn1 -- LeftHipRollLink/RConn1 -- Motor 2 - HipRoll/RConn1
  LeftFootTf/LConn1 -- LeftAnkleRollLink/RConn1 -- Motor6 - AnkleRoll/RConn1
  LeftKneeTf_A/LConn1 -- LeftHipPitchLink_1/RConn1 -- Motor 3_1 - HipPitch/RConn1
  LeftAnklePitch/RConn1 -- Motor5 - AnklePitch/LConn1
  Motor4_1 - KneePitch/LConn1 -- LeftKneeTf_A/RConn1
  LeftHipYawTf/RConn1 -- Motor 1 - HipYaw/LConn1
  LeftAnklePitch/LConn1 -- LeftKneeTf_1/RConn1 -- LeftKneeTf_2/RConn1
  FootContact/LConn1 -- LeftFootTf/RConn1
  LeftHipYawLink/RConn1 -- LeftHipRollTf/LConn1 -- Motor 1 - HipYaw/RConn1
  FootContact/RConn1 -- Foot sole CF/RConn1
  LeftHipYawTf/LConn1 -- Mechanical connection/RConn1
  LeftHipPitchTf_1/RConn1 -- Motor 3_1 - HipPitch/LConn1
  LeftHipPitchTf_2/RConn1 -- Motor 3_2 - HipPitch/LConn1
  LeftKneeTf_B/LConn1 -- LeftHipPitchLink_2/RConn1 -- Motor 3_2 - HipPitch/RConn1
  Motor 4_2 - KneePitch/RConn1 -- LeftKneeTf_2/LConn1
  Motor 4_2 - KneePitch/LConn1 -- LeftKneeTf_B/RConn1
  LeftKneeLink/RConn1 -- Motor4_1 - KneePitch/RConn1 -- LeftGasDamper/RConn1 -- LeftKneeTf_1/LConn1
  LEFT: dyn. ref. link 1/LConn1 -- LeftHipYawLink/LConn1
  LEFT: dyn. ref. link 2/LConn1 -- LeftHipRollLink/LConn1
  LEFT: dyn. ref. link 4/LConn1 -- LeftKneeLink/LConn1
  LEFT: dyn. ref. link 5/LConn1 -- LeftAnklePitchLink/LConn1
  LEFT: dyn. ref. link 6/LConn1 -- LeftAnkleRollLink/LConn1
  LeftHipPitchLink_1/LConn1 -- LEFT: dyn. ref. link 3_1/LConn1
  LEFT: dyn. ref. link 3_2/LConn1 -- LeftHipPitchLink_2/LConn1

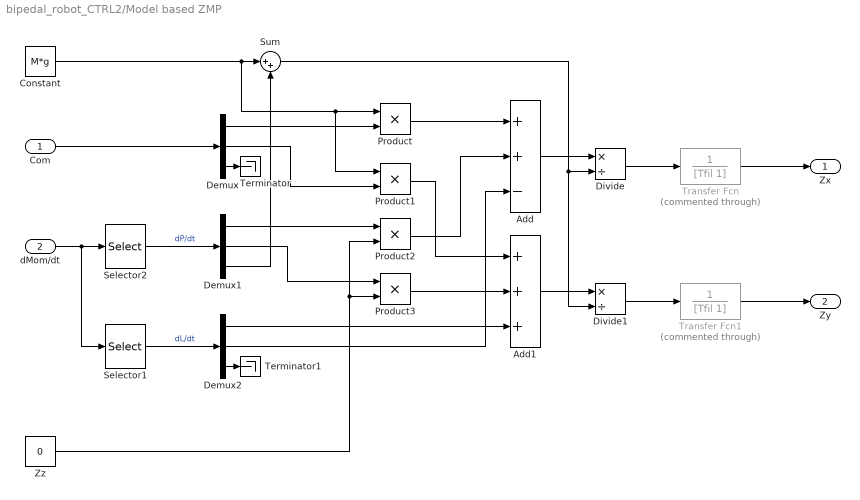
== system bipedal_robot_CTRL2/Model based ZMP ==
  Com : Inport
  dMom/dt : Inport  Port=2
  Add : Sum  Inputs=++-
  Add1 : Sum  Inputs=+++
  Constant : Constant  Value=M*g
  Demux : Demux  Outputs=3
  Demux1 : Demux  Outputs=3
  Demux2 : Demux  Outputs=3
  Divide : Product  Inputs=*/
  Divide1 : Product  Inputs=*/
  Product{,1..3} (4 alike) : Product
  Selector1 : Selector  InputPortWidth=6  IndexOptions=Index vector (dialog)  Indices=[4:6]  OutputSizes=1
  Selector2 : Selector  InputPortWidth=6  IndexOptions=Index vector (dialog)  Indices=[1:3]  OutputSizes=1
  Sum : Sum  Inputs=|++
  Terminator : Terminator
  Terminator1 : Terminator
  Transfer Fcn : TransferFcn  Commented=through  Denominator=[Tfil 1]
  Transfer Fcn1 : TransferFcn  Commented=through  Denominator=[Tfil 1]
  Zz : Constant  Value=0
  Zx : Outport
  Zy : Outport  Port=2
  wires:
  Com/1 -> Demux/1
  dMom/dt/1 -> Selector1/1, Selector2/1
  Selector1/1 -> Demux2/1  "dL/dt"
  Demux/1 -> Product/2
  Constant/1 -> Sum/1, Product1/1, Product/1
  Demux/2 -> Product1/2
  Demux1/1 -> Product2/1
  Zz/1 -> Product3/2, Product2/2
  Demux1/2 -> Product3/1
  Demux1/3 -> Sum/2
  Demux2/3 -> Terminator1/1
  Demux/3 -> Terminator/1
  Product/1 -> Add/1
  Product2/1 -> Add/2
  Demux2/2 -> Add/3
  Demux2/1 -> Add1/3
  Product3/1 -> Add1/2
  Product1/1 -> Add1/1
  Add/1 -> Divide/1
  Add1/1 -> Divide1/1
  Sum/1 -> Divide1/2, Divide/2
  Divide/1 -> Transfer Fcn/1
  Divide1/1 -> Transfer Fcn1/1
  Selector2/1 -> Demux1/1  "dP/dt"
  Transfer Fcn1/1 -> Zy/1
  Transfer Fcn/1 -> Zx/1
